simulink model "sampleModel196"  (Simulink 9.1)
settings: Solver=VariableStepAuto  StartTime=0.0  StopTime=10.0  RelTol=1e-3
undefined symbols (not defined in the file): DiscIntNeverNeededParam, Newton, Raphson
libraries: simulink x17
settings Model: Creator=DELL  LastModifiedBy=DELL
settings DataIOCC: SaveFormat=Dataset
settings OptimizationCC: LifeSpan=auto
settings DebuggingCC: UnderspecifiedInitializationDetection=Simplified  MergeDetectMultiDrivingBlocksExec=error  SFUnexpectedBacktrackingDiag=error  SFNoUnconditionalDefaultTransitionDiag=error  SFExecutionAtInitializationDiag=warning
settings HardwareCC: ProdBitPerPointer=64  ProdBitPerSizeT=64  ProdBitPerPtrDiffT=64  ProdLargestAtomicFloat=Float  ProdIntDivRoundTo=Zero  ProdEndianess=LittleEndian  ProdWordSize=64  ProdHWDeviceType=Intel->x86-64 (Windows64)
settings ModelReferenceCC: PropagateSignalLabelsOutOfModel=on
settings CodeAppCC: StateflowObjectComments=off
settings GRTTargetCC: TargetLangStandard=C99 (ISO)  CombineOutputUpdateFcns=on  GRTInterface=off
settings ConfigComp: CovMetricSettings=dwe  CovHtmlReporting=off  CovSaveCumulativeToWorkspaceVar=off  CovSaveSingleToWorkspaceVar=off  CovExternalEMLEnable=on

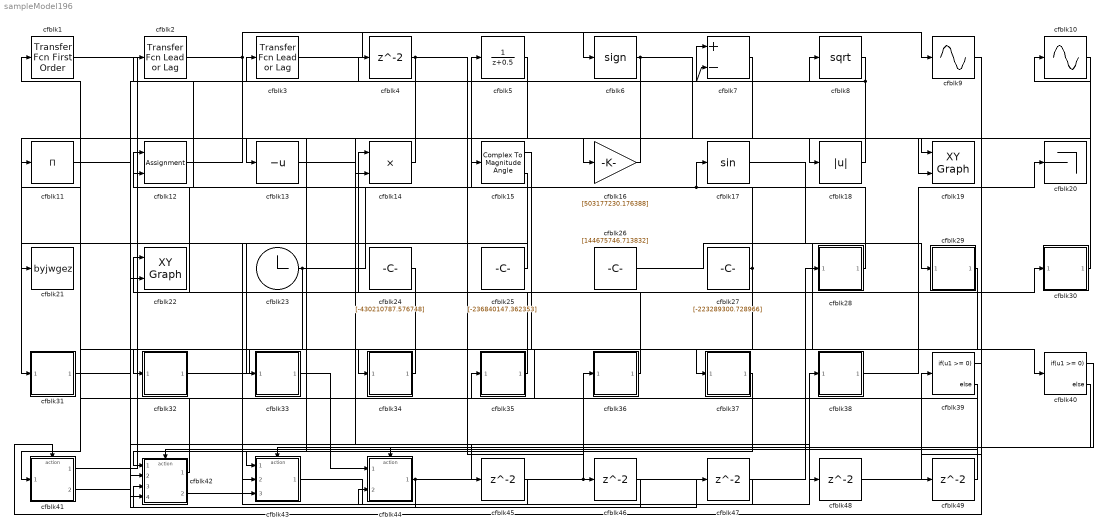
== system sampleModel196 ==
  cfblk1 : simulink/Discrete/Transfer Fcn First Order  PoleZ=0.95  ICPrevOutput=0.0  DoSatur=off
      settings: SourceProductName=Simulink
  cfblk10 : Sin  TimeSource=Use external signal  SampleTime=0
  cfblk11 : Product  Inputs=*
  cfblk12 : Assignment  DiagnosticForDimensions=Warning  IndexOptions=Index vector (dialog)  Indices=1  OutputSizes=1
  cfblk13 : UnaryMinus
  cfblk14 : Product  Inputs=**
  cfblk15 : ComplexToMagnitudeAngle
  cfblk16 : Gain  Gain=[503177230.176388]
  cfblk17 : Trigonometry
  cfblk18 : Abs
  cfblk19 : simulink/Sinks/XY Graph  xmin=-1  xmax=1  ymin=-1  ymax=1  st=-1
  cfblk2 : simulink/Discrete/Transfer Fcn Lead or Lag  PoleZ=0.95  ZeroZ=0.75  ICPrevOutput=0.0  ICPrevInput=0.0  DoSatur=off
      settings: SourceProductName=Simulink  SourceProductBaseCode=SL
  cfblk20 : Terminator
  cfblk21 : ToWorkspace  VariableName=byjwgez  SaveFormat=Timeseries  SampleTime=-1
  cfblk22 : simulink/Sinks/XY Graph  xmin=-1  xmax=1  ymin=-1  ymax=1  st=-1
  cfblk23 : Clock
  cfblk24 : Constant  Value=[-430210787.576748]  SampleTime=1
  cfblk25 : Constant  Value=[-236840147.362353]  SampleTime=1
  cfblk26 : Constant  Value=[144675746.713832]  SampleTime=1
  cfblk27 : Constant  Value=[-223289300.728966]  SampleTime=1
  cfblk28 : Subsystem
  cfblk29 : Subsystem
  cfblk3 : simulink/Discrete/Transfer Fcn Lead or Lag  PoleZ=0.95  ZeroZ=0.75  ICPrevOutput=0.0  ICPrevInput=0.0  DoSatur=off
      settings: SourceProductName=Simulink  SourceProductBaseCode=SL
  cfblk30 : Subsystem
  cfblk31 : Subsystem
  cfblk32 : Subsystem
  cfblk33 : Subsystem
  cfblk34 : Subsystem
  cfblk35 : Subsystem
  cfblk36 : Subsystem
  cfblk37 : Subsystem
  cfblk38 : Subsystem
  cfblk39 : If  IfExpression=u1 >= 0  SampleTime=1
  cfblk{4,45..49} (6 alike) : Delay  SampleTime=1
  cfblk40 : If  IfExpression=u1 >= 0  SampleTime=1
  cfblk41 : Subsystem  TreatAsAtomicUnit=on
  cfblk42 : Subsystem  TreatAsAtomicUnit=on
  cfblk43 : Subsystem  TreatAsAtomicUnit=on
  cfblk44 : Subsystem  TreatAsAtomicUnit=on
  cfblk5 : DiscreteTransferFcn  SampleTime=1
  cfblk6 : Signum
  cfblk7 : Sum  Inputs=+-
  cfblk8 : Sqrt  SaturateOnIntegerOverflow=on
  cfblk9 : Sin  TimeSource=Use external signal  SampleTime=0
  wires:
  cfblk33/1(cfblk2) -> cfblk44/1(cfblk1)
  cfblk15/1 -> cfblk34/1(cfblk1)
  cfblk43/1(cfblk2) -> cfblk38/1(cfblk1)
  cfblk27/1 -> cfblk35/1(cfblk1), cfblk12/2
  cfblk28/1(cfblk2) -> cfblk17/1, cfblk2/1
  cfblk26/1 -> cfblk40/1
  cfblk41/1(cfblk2) -> cfblk8/1
  cfblk23/1 -> cfblk5/1, cfblk42/4(cfblk13)
  cfblk8/1 -> cfblk18/1, cfblk7/2
  cfblk14/1 -> cfblk3/1
  cfblk6/1 -> cfblk13/1, cfblk19/2
  cfblk18/1 -> cfblk16/1
  cfblk17/1 -> cfblk29/1(cfblk1)
  cfblk4/1 -> cfblk31/1(cfblk1), cfblk46/1
  cfblk2/1 -> cfblk9/1, cfblk19/1
  cfblk3/1 -> cfblk6/1
  cfblk12/1 -> cfblk15/1
  cfblk16/1 -> cfblk4/1
  cfblk24/1 -> cfblk41/1(cfblk1)
  cfblk38/1(cfblk2) -> cfblk20/1
  cfblk5/1 -> cfblk43/1(cfblk1)
  cfblk30/1(cfblk2) -> cfblk10/1
  cfblk32/1(cfblk2) -> cfblk37/1(cfblk1)
  cfblk37/1(cfblk2) -> cfblk42/1(cfblk1)
  cfblk29/1(cfblk2) -> cfblk32/1(cfblk1)
  cfblk25/1 -> cfblk21/1
  cfblk34/1(cfblk2) -> cfblk22/1
  cfblk15/2 -> cfblk43/3(cfblk9)
  cfblk36/1(cfblk2) -> cfblk14/1
  cfblk7/1 -> cfblk22/2
  cfblk31/1(cfblk2) -> cfblk7/1
  cfblk44/1(cfblk2) -> cfblk28/1(cfblk1), cfblk36/1(cfblk1), cfblk42/3(cfblk12)
  cfblk10/1 -> cfblk14/2
  cfblk42/1(cfblk2) -> cfblk11/1
  cfblk42/2(cfblk14) -> cfblk30/1(cfblk1)
  cfblk1/1 -> cfblk33/1(cfblk1)
  cfblk35/1(cfblk2) -> cfblk12/1
  cfblk39/1 -> cfblk41/Action
  cfblk39/2 -> cfblk42/Action
  cfblk40/1 -> cfblk43/Action
  cfblk40/2 -> cfblk44/Action
  cfblk11/1 -> cfblk45/1
  cfblk45/1 -> cfblk43/2(cfblk8)
  cfblk46/1 -> cfblk42/2(cfblk11)
  cfblk41/2(cfblk13) -> cfblk47/1
  cfblk47/1 -> cfblk44/2(cfblk14)
  cfblk13/1 -> cfblk48/1
  cfblk48/1 -> cfblk39/1
  cfblk9/1 -> cfblk49/1
  cfblk49/1 -> cfblk1/1

== system sampleModel196/cfblk28 ==
  cfblk1 : Inport
  cfblk2 : Outport
  wires:
  cfblk1/1 -> cfblk2/1

== system sampleModel196/cfblk29 ==
  cfblk1 : Inport
  cfblk2 : Outport
  wires:
  cfblk1/1 -> cfblk2/1

== system sampleModel196/cfblk30 ==
  cfblk1 : Inport
  cfblk2 : Outport
  wires:
  cfblk1/1 -> cfblk2/1

== system sampleModel196/cfblk31 ==
  cfblk1 : Inport
  cfblk2 : Outport
  wires:
  cfblk1/1 -> cfblk2/1

== system sampleModel196/cfblk32 ==
  cfblk1 : Inport
  cfblk2 : Outport
  wires:
  cfblk1/1 -> cfblk2/1

== system sampleModel196/cfblk33 ==
  cfblk1 : Inport
  cfblk2 : Outport
  wires:
  cfblk1/1 -> cfblk2/1

== system sampleModel196/cfblk34 ==
  cfblk1 : Inport
  cfblk2 : Outport
  wires:
  cfblk1/1 -> cfblk2/1

== system sampleModel196/cfblk35 ==
  cfblk1 : Inport
  cfblk2 : Outport
  wires:
  cfblk1/1 -> cfblk2/1

== system sampleModel196/cfblk36 ==
  cfblk1 : Inport
  cfblk2 : Outport
  wires:
  cfblk1/1 -> cfblk2/1

== system sampleModel196/cfblk37 ==
  cfblk1 : Inport
  cfblk2 : Outport
  wires:
  cfblk1/1 -> cfblk2/1

== system sampleModel196/cfblk38 ==
  cfblk1 : Inport
  cfblk2 : Outport
  wires:
  cfblk1/1 -> cfblk2/1

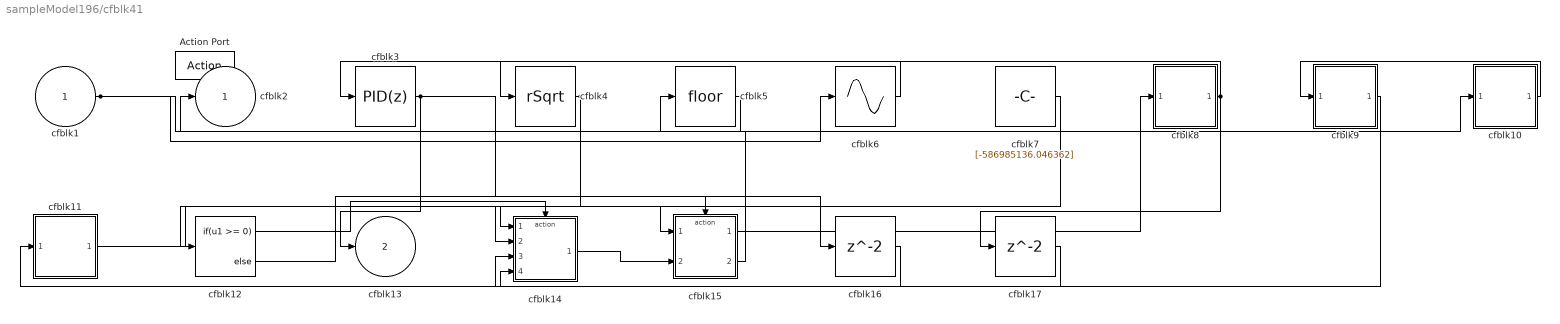
== system sampleModel196/cfblk41 ==
  cfblk1 : Inport
  Action Port : ActionPort  ActionType=then
  cfblk10 : Subsystem
  cfblk11 : Subsystem
  cfblk12 : If  IfExpression=u1 >= 0  SampleTime=1
  cfblk14 : Subsystem  TreatAsAtomicUnit=on
  cfblk15 : Subsystem  TreatAsAtomicUnit=on
  cfblk16 : Delay
  cfblk17 : Delay
  cfblk3 : simulink/Continuous/PID Controller  Controller=PID  TimeDomain=Discrete-time  SampleTime=-1  IntegratorMethod=Forward Euler  FilterMethod=Forward Euler  Form=Parallel  UseFilter=on  ControllerParametersSource=internal  P=1  I=1  D=0  N=100  InitialConditionSource=internal  InitialConditionForIntegrator=0  InitialConditionForFilter=0  ExternalReset=none  LimitOutput=off  UpperSaturationLimit=inf  LowerSaturationLimit=-inf  LinearizeAsGain=off  AntiWindupMode=none  Kb=1  TrackingMode=off  Kt=1  PParamMin=[]  PParamMax=[]  IParamMin=[]  IParamMax=[]  DParamMin=[]  DParamMax=[]  NParamMin=[]  NParamMax=[]  KbParamMin=[]  KbParamMax=[]  KtParamMin=[]  KtParamMax=[]  POutMin=[]  POutMax=[]  IOutMin=[]  IOutMax=[]  DOutMin=[]  DOutMax=[]  NOutMin=[]  NOutMax=[]  KbOutMin=[]  KbOutMax=[]  KtOutMin=[]  KtOutMax=[]  IntegratorOutMin=[]  IntegratorOutMax=[]  FilterOutMin=[]  FilterOutMax=[]  SumOutMin=[]  SumOutMax=[]  SumI1OutMin=[]  SumI1OutMax=[]  SumI2OutMin=[]  SumI2OutMax=[]  SumI3OutMin=[]  SumI3OutMax=[]  SumDOutMin=[]  SumDOutMax=[]  SaturationOutMin=[]  SaturationOutMax=[]  IntegratorContinuousStateAttributes=''  IntegratorStateMustResolveToSignalObject=off  IntegratorRTWStateStorageClass=Auto  FilterContinuousStateAttributes=''  FilterStateMustResolveToSignalObject=off  FilterRTWStateStorageClass=Auto  DifferentiatorICPrevScaledInput=0  DifferentiatorOutMin=[]  DifferentiatorOutMax=[]  FilterDiffOutCoefMin=[]  FilterDiffOutCoefMax=[]  SumDenOutMin=[]  SumDenOutMax=[]  SumNumOutMin=[]  SumNumOutMax=[]  ReciprocalOutMin=[]  ReciprocalOutMax=[]  DivideOutMin=[]  DivideOutMax=[]  TunerSelectOption=Transfer Function Based (PID Tuner App)
  cfblk4 : Sqrt  Operator=rSqrt  AlgorithmType=Newton-Raphson  SaturateOnIntegerOverflow=on
  cfblk5 : Rounding
  cfblk6 : Sin  TimeSource=Use external signal  SampleTime=0
  cfblk7 : Constant  Value=[-586985136.046362]  SampleTime=1
  cfblk8 : Subsystem
  cfblk9 : Subsystem
  cfblk2 : Outport
  cfblk13 : Outport  Port=2
  wires:
  cfblk15/1(cfblk2) -> cfblk8/1(cfblk1)
  cfblk8/1(cfblk2) -> cfblk3/1, cfblk17/1
  cfblk5/1 -> cfblk2/1
  cfblk9/1(cfblk2) -> cfblk11/1(cfblk1)
  cfblk11/1(cfblk2) -> cfblk15/1(cfblk1)
  cfblk7/1 -> cfblk14/1(cfblk1)
  cfblk1/1 -> cfblk6/1, cfblk10/1(cfblk1)
  cfblk3/1 -> cfblk13/1, cfblk16/1
  cfblk4/1 -> cfblk12/1, cfblk14/2(cfblk11)
  cfblk6/1 -> cfblk4/1
  cfblk10/1(cfblk2) -> cfblk9/1(cfblk1)
  cfblk15/2(cfblk9) -> cfblk5/1
  cfblk14/1(cfblk2) -> cfblk15/2(cfblk8)
  cfblk12/1 -> cfblk14/Action
  cfblk12/2 -> cfblk15/Action
  cfblk16/1 -> cfblk14/4(cfblk13)
  cfblk17/1 -> cfblk14/3(cfblk12)

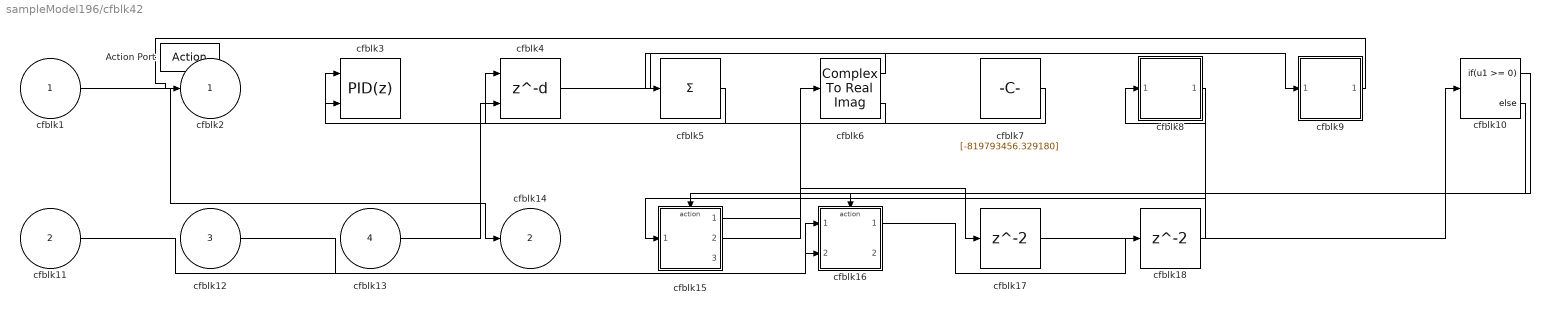
== system sampleModel196/cfblk42 ==
  cfblk1 : Inport
  cfblk11 : Inport  Port=2
  cfblk12 : Inport  Port=3
  cfblk13 : Inport  Port=4
  Action Port : ActionPort  ActionType=else
  cfblk10 : If  IfExpression=u1 >= 0  SampleTime=1
  cfblk15 : Subsystem  TreatAsAtomicUnit=on
  cfblk16 : Subsystem  TreatAsAtomicUnit=on
  cfblk17 : Delay
  cfblk18 : Delay
  cfblk3 : simulink/Continuous/PID Controller (2DOF)  Controller=PID  TimeDomain=Discrete-time  SampleTime=-1  IntegratorMethod=Forward Euler  FilterMethod=Forward Euler  Form=Parallel  UseFilter=on  ControllerParametersSource=internal  P=1  I=1  D=0  N=100  b=1  c=1  InitialConditionSource=internal  InitialConditionForIntegrator=0  InitialConditionForFilter=0  ExternalReset=none  LimitOutput=off  UpperSaturationLimit=inf  LowerSaturationLimit=-inf  LinearizeAsGain=off  AntiWindupMode=none  Kb=1  TrackingMode=off  Kt=1  PParamMin=[]  PParamMax=[]  IParamMin=[]  IParamMax=[]  DParamMin=[]  DParamMax=[]  NParamMin=[]  NParamMax=[]  bParamMin=[]  bParamMax=[]  cParamMin=[]  cParamMax=[]  KbParamMin=[]  KbParamMax=[]  KtParamMin=[]  KtParamMax=[]  POutMin=[]  POutMax=[]  IOutMin=[]  IOutMax=[]  DOutMin=[]  DOutMax=[]  NOutMin=[]  NOutMax=[]  bOutMin=[]  bOutMax=[]  cOutMin=[]  cOutMax=[]  KbOutMin=[]  KbOutMax=[]  KtOutMin=[]  KtOutMax=[]  IntegratorOutMin=[]  IntegratorOutMax=[]  FilterOutMin=[]  FilterOutMax=[]  SumOutMin=[]  SumOutMax=[]  Sum1OutMin=[]  Sum1OutMax=[]  Sum2OutMin=[]  Sum2OutMax=[]  Sum3OutMin=[]  Sum3OutMax=[]  SumI1OutMin=[]  SumI1OutMax=[]  SumI2OutMin=[]  SumI2OutMax=[]  SumI3OutMin=[]  SumI3OutMax=[]  SumDOutMin=[]  SumDOutMax=[]  SaturationOutMin=[]  SaturationOutMax=[]  IntegratorContinuousStateAttributes=''  IntegratorStateMustResolveToSignalObject=off  IntegratorRTWStateStorageClass=Auto  FilterContinuousStateAttributes=''  FilterStateMustResolveToSignalObject=off  FilterRTWStateStorageClass=Auto  DifferentiatorICPrevScaledInput=0  DifferentiatorOutMin=[]  DifferentiatorOutMax=[]  FilterDiffOutCoefMin=[]  FilterDiffOutCoefMax=[]  SumDenOutMin=[]  SumDenOutMax=[]  SumNumOutMin=[]  SumNumOutMax=[]  ReciprocalOutMin=[]  ReciprocalOutMax=[]  DivideOutMin=[]  DivideOutMax=[]  TunerSelectOption=Transfer Function Based (PID Tuner App)
  cfblk4 : Delay  DelayLengthSource=Input port
      settings: InputPortMap=u0,p1
  cfblk5 : Sum  Inputs=+
  cfblk6 : ComplexToRealImag
  cfblk7 : Constant  Value=[-819793456.329180]  SampleTime=1
  cfblk8 : Subsystem
  cfblk9 : Subsystem
  cfblk2 : Outport
  cfblk14 : Outport  Port=2
  wires:
  cfblk4/1 -> cfblk9/1(cfblk1)
  cfblk1/1 -> cfblk14/1
  cfblk11/1 -> cfblk16/1(cfblk1)
  cfblk7/1 -> cfblk4/1
  cfblk9/1(cfblk2) -> cfblk2/1
  cfblk12/1 -> cfblk16/2(cfblk11)
  cfblk6/1 -> cfblk5/1
  cfblk13/1 -> cfblk4/2
  cfblk8/1(cfblk2) -> cfblk15/1(cfblk1)
  cfblk6/2 -> cfblk3/1
  cfblk15/2(cfblk16) -> cfblk6/1
  cfblk5/1 -> cfblk3/2
  cfblk10/1 -> cfblk15/Action
  cfblk10/2 -> cfblk16/Action
  cfblk15/1(cfblk2) -> cfblk17/1
  cfblk17/1 -> cfblk10/1
  cfblk16/1(cfblk2) -> cfblk18/1
  cfblk18/1 -> cfblk8/1(cfblk1)

== system sampleModel196/cfblk43 ==
  cfblk1 : Inport
  cfblk8 : Inport  Port=2
  cfblk9 : Inport  Port=3
  Action Port : ActionPort  ActionType=then
  cfblk3 : DiscreteStateSpace  SampleTime=-1
  cfblk4 : DiscreteFilter
  cfblk5 : DiscreteZeroPole  Poles=[0 0.5]  Gain=1  SampleTime=-1
  cfblk6 : Constant  Value=[-475565543.118266]  SampleTime=1
  cfblk7 : Subsystem
  cfblk2 : Outport
  wires:
  cfblk4/1 -> cfblk2/1
  cfblk6/1 -> cfblk4/1
  cfblk8/1 -> cfblk5/1
  cfblk5/1 -> cfblk7/1(cfblk1)
  cfblk7/1(cfblk2) -> cfblk3/1

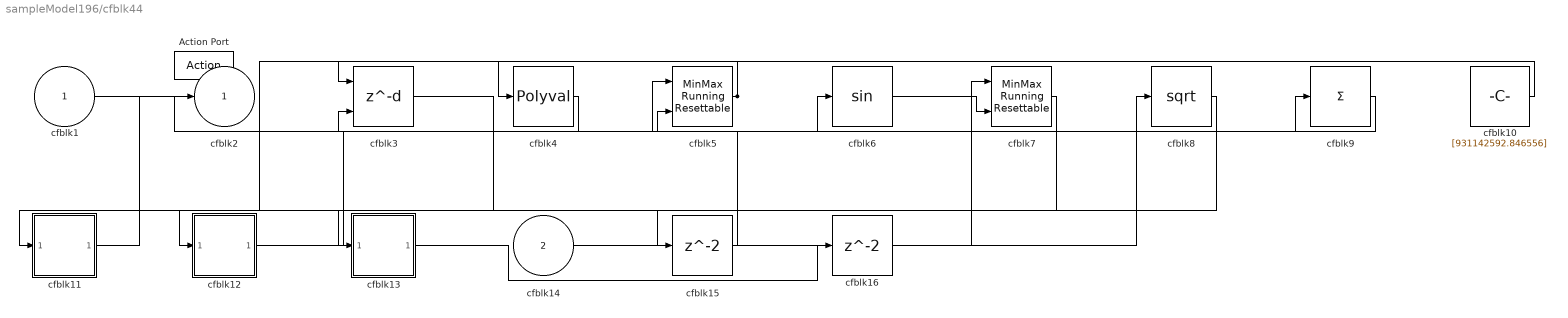
== system sampleModel196/cfblk44 ==
  cfblk1 : Inport
  cfblk14 : Inport  Port=2
  Action Port : ActionPort  ActionType=else
  cfblk10 : Constant  Value=[931142592.846556]  SampleTime=1
  cfblk11 : Subsystem
  cfblk12 : Subsystem
  cfblk13 : Subsystem
  cfblk15 : Delay
  cfblk16 : Delay
  cfblk3 : Delay  DelayLengthSource=Input port
      settings: InputPortMap=u0,p1
  cfblk4 : Polyval  Coefs=[ +2.081618890e-019, -1.441693666e-014, +4.719686976e-010, -8.536869453e-006, +1.621573104e-001, -8.087801117e+001 ]
  cfblk5 : simulink/Math Operations/MinMax Running Resettable  Function=min  vinit=0.0
  cfblk6 : Trigonometry
  cfblk7 : simulink/Math Operations/MinMax Running Resettable  Function=min  vinit=0.0
  cfblk8 : Sqrt  SaturateOnIntegerOverflow=on
  cfblk9 : Sum  Inputs=+
  cfblk2 : Outport
  wires:
  cfblk12/1(cfblk2) -> cfblk6/1
  cfblk10/1 -> cfblk12/1(cfblk1)
  cfblk11/1(cfblk2) -> cfblk2/1
  cfblk1/1 -> cfblk9/1
  cfblk14/1 -> cfblk8/1
  cfblk5/1 -> cfblk3/1, cfblk4/1
  cfblk9/1 -> cfblk5/2
  cfblk4/1 -> cfblk3/2
  cfblk7/1 -> cfblk13/1(cfblk1)
  cfblk6/1 -> cfblk7/2
  cfblk8/1 -> cfblk11/1(cfblk1)
  cfblk3/1 -> cfblk15/1
  cfblk15/1 -> cfblk5/1
  cfblk13/1(cfblk2) -> cfblk16/1
  cfblk16/1 -> cfblk7/1

== system sampleModel196/cfblk41/cfblk10 ==
  cfblk1 : Inport
  cfblk2 : Outport
  wires:
  cfblk1/1 -> cfblk2/1

== system sampleModel196/cfblk41/cfblk11 ==
  cfblk1 : Inport
  cfblk2 : Outport
  wires:
  cfblk1/1 -> cfblk2/1

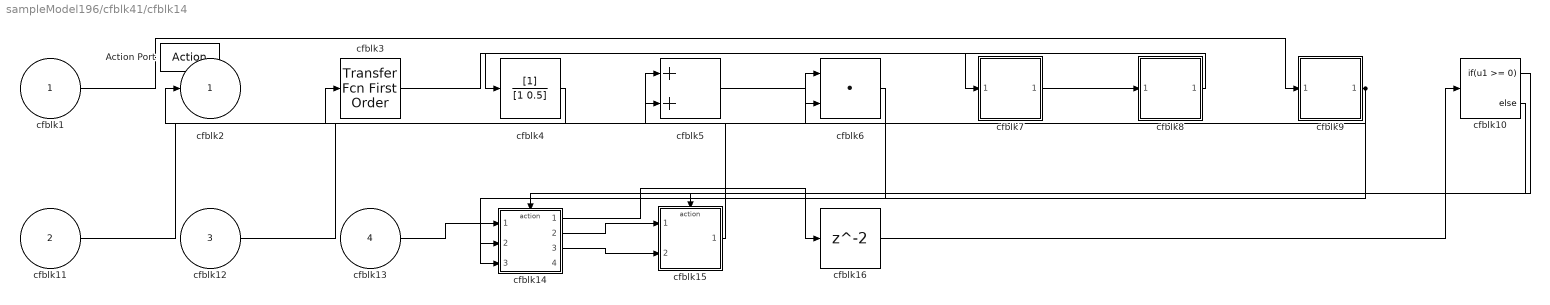
== system sampleModel196/cfblk41/cfblk14 ==
  cfblk1 : Inport
  cfblk11 : Inport  Port=2
  cfblk12 : Inport  Port=3
  cfblk13 : Inport  Port=4
  Action Port : ActionPort  ActionType=then
  cfblk10 : If  IfExpression=u1 >= 0  SampleTime=1
  cfblk14 : Subsystem  TreatAsAtomicUnit=on
  cfblk15 : Subsystem  TreatAsAtomicUnit=on
  cfblk16 : Delay
  cfblk3 : simulink/Discrete/Transfer Fcn First Order  PoleZ=0.95  ICPrevOutput=0.0  DoSatur=off
      settings: SourceProductName=Simulink
  cfblk4 : DiscreteFilter
  cfblk5 : Sum
  cfblk6 : DotProduct  InputSameDT=on  OutDataTypeStr=Inherit: Inherit via internal rule
  cfblk7 : Subsystem
  cfblk8 : Subsystem
  cfblk9 : Subsystem
  cfblk2 : Outport
  wires:
  cfblk8/1(cfblk2) -> cfblk4/1
  cfblk11/1 -> cfblk6/1
  cfblk1/1 -> cfblk9/1(cfblk1)
  cfblk12/1 -> cfblk5/1
  cfblk15/1(cfblk2) -> cfblk3/1
  cfblk3/1 -> cfblk7/1(cfblk1)
  cfblk9/1(cfblk2) -> cfblk5/2, cfblk14/3(cfblk13)
  cfblk5/1 -> cfblk6/2
  cfblk7/1(cfblk2) -> cfblk8/1(cfblk1)
  cfblk13/1 -> cfblk14/1(cfblk1)
  cfblk4/1 -> cfblk2/1
  cfblk6/1 -> cfblk14/2(cfblk12)
  cfblk14/2(cfblk14) -> cfblk15/1(cfblk1)
  cfblk14/3(cfblk15) -> cfblk15/2(cfblk16)
  cfblk10/1 -> cfblk14/Action
  cfblk10/2 -> cfblk15/Action
  cfblk14/1(cfblk2) -> cfblk16/1
  cfblk16/1 -> cfblk10/1

== system sampleModel196/cfblk41/cfblk15 ==
  cfblk1 : Inport
  cfblk8 : Inport  Port=2
  Action Port : ActionPort  ActionType=else
  cfblk3 : DiscreteFir
  cfblk4 : simulink/Discrete/Difference  ICPrevInput=0.0  OutMin=[]  OutMax=[]  OutDataTypeStr=Inherit: Inherit via back propagation  OutDataType=fixdt(1, 16)  OutScaling=2^-10  DoSatur=off
  cfblk5 : Constant  Value=[-973339246.254504]  SampleTime=1
  cfblk6 : Constant  Value=[-836028439.478681]  SampleTime=1
  cfblk7 : Constant  Value=[-477392529.505172]  SampleTime=1
  cfblk2 : Outport
  cfblk9 : Outport  Port=2
  wires:
  cfblk7/1 -> cfblk3/1
  cfblk8/1 -> cfblk4/1
  cfblk1/1 -> cfblk2/1
  cfblk3/1 -> cfblk9/1

== system sampleModel196/cfblk41/cfblk8 ==
  cfblk1 : Inport
  cfblk2 : Outport
  wires:
  cfblk1/1 -> cfblk2/1

== system sampleModel196/cfblk41/cfblk9 ==
  cfblk1 : Inport
  cfblk2 : Outport
  wires:
  cfblk1/1 -> cfblk2/1

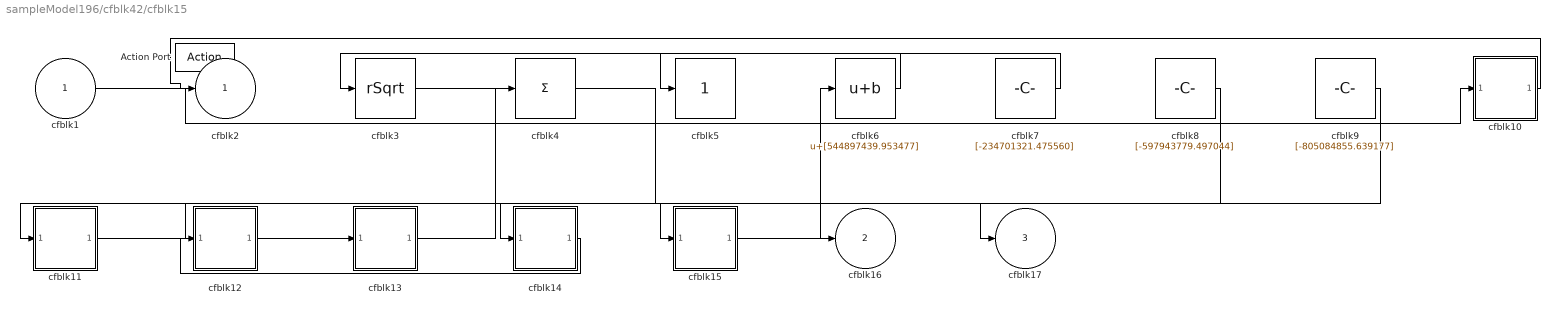
== system sampleModel196/cfblk42/cfblk15 ==
  cfblk1 : Inport
  Action Port : ActionPort  ActionType=then
  cfblk10 : Subsystem
  cfblk11 : Subsystem
  cfblk12 : Subsystem
  cfblk13 : Subsystem
  cfblk14 : Subsystem
  cfblk15 : Subsystem
  cfblk3 : Sqrt  Operator=rSqrt  AlgorithmType=Newton-Raphson  SaturateOnIntegerOverflow=on
  cfblk4 : Sum  Inputs=+
  cfblk5 : simulink/Math Operations/Slider Gain  gain=1  low=0  high=2
  cfblk6 : Bias  Bias=[544897439.953477]
  cfblk7 : Constant  Value=[-234701321.475560]  SampleTime=1
  cfblk8 : Constant  Value=[-597943779.497044]  SampleTime=1
  cfblk9 : Constant  Value=[-805084855.639177]  SampleTime=1
  cfblk2 : Outport
  cfblk16 : Outport  Port=2
  cfblk17 : Outport  Port=3
  wires:
  cfblk1/1 -> cfblk10/1(cfblk1)
  cfblk8/1 -> cfblk14/1(cfblk1)
  cfblk15/1(cfblk2) -> cfblk6/1
  cfblk7/1 -> cfblk3/1
  cfblk13/1(cfblk2) -> cfblk4/1
  cfblk11/1(cfblk2) -> cfblk16/1
  cfblk14/1(cfblk2) -> cfblk12/1(cfblk1)
  cfblk10/1(cfblk2) -> cfblk2/1
  cfblk12/1(cfblk2) -> cfblk13/1(cfblk1)
  cfblk6/1 -> cfblk5/1
  cfblk4/1 -> cfblk17/1
  cfblk9/1 -> cfblk11/1(cfblk1)
  cfblk3/1 -> cfblk15/1(cfblk1)

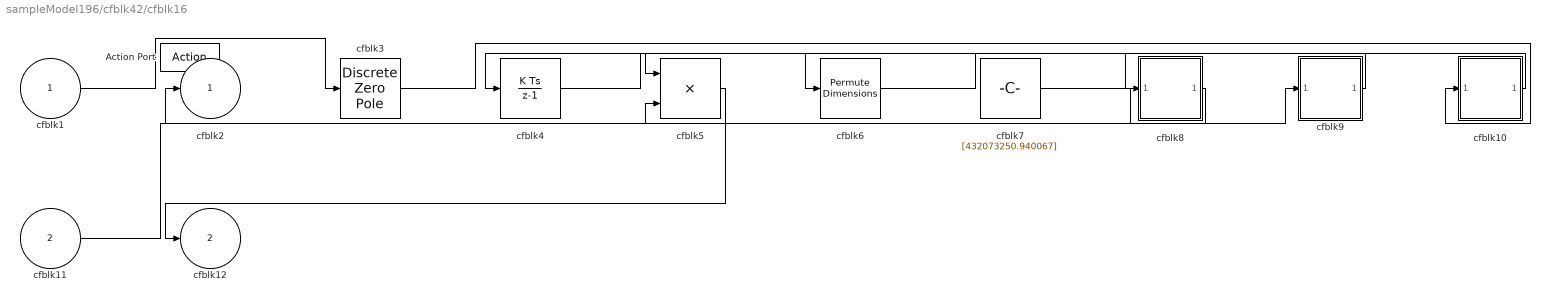
== system sampleModel196/cfblk42/cfblk16 ==
  cfblk1 : Inport
  cfblk11 : Inport  Port=2
  Action Port : ActionPort  ActionType=else
  cfblk10 : Subsystem
  cfblk3 : DiscreteZeroPole  Poles=[0 0.5]  Gain=1  SampleTime=-1
  cfblk4 : DiscreteIntegrator  SampleTime=-1  ICPrevOutput=DiscIntNeverNeededParam  ICPrevScaledInput=DiscIntNeverNeededParam
  cfblk5 : Product
  cfblk6 : PermuteDimensions
  cfblk7 : Constant  Value=[432073250.940067]  SampleTime=1
  cfblk8 : Subsystem
  cfblk9 : Subsystem
  cfblk2 : Outport
  cfblk12 : Outport  Port=2
  wires:
  cfblk5/1 -> cfblk12/1
  cfblk10/1(cfblk2) -> cfblk4/1
  cfblk7/1 -> cfblk9/1(cfblk1)
  cfblk9/1(cfblk2) -> cfblk5/1
  cfblk8/1(cfblk2) -> cfblk2/1
  cfblk1/1 -> cfblk3/1
  cfblk11/1 -> cfblk5/2
  cfblk3/1 -> cfblk10/1(cfblk1)
  cfblk6/1 -> cfblk8/1(cfblk1)
  cfblk4/1 -> cfblk6/1

== system sampleModel196/cfblk42/cfblk8 ==
  cfblk1 : Inport
  cfblk2 : Outport
  wires:
  cfblk1/1 -> cfblk2/1

== system sampleModel196/cfblk42/cfblk9 ==
  cfblk1 : Inport
  cfblk2 : Outport
  wires:
  cfblk1/1 -> cfblk2/1

== system sampleModel196/cfblk43/cfblk7 ==
  cfblk1 : Inport
  cfblk2 : Outport
  wires:
  cfblk1/1 -> cfblk2/1

== system sampleModel196/cfblk44/cfblk11 ==
  cfblk1 : Inport
  cfblk2 : Outport
  wires:
  cfblk1/1 -> cfblk2/1

== system sampleModel196/cfblk44/cfblk12 ==
  cfblk1 : Inport
  cfblk2 : Outport
  wires:
  cfblk1/1 -> cfblk2/1

== system sampleModel196/cfblk44/cfblk13 ==
  cfblk1 : Inport
  cfblk2 : Outport
  wires:
  cfblk1/1 -> cfblk2/1

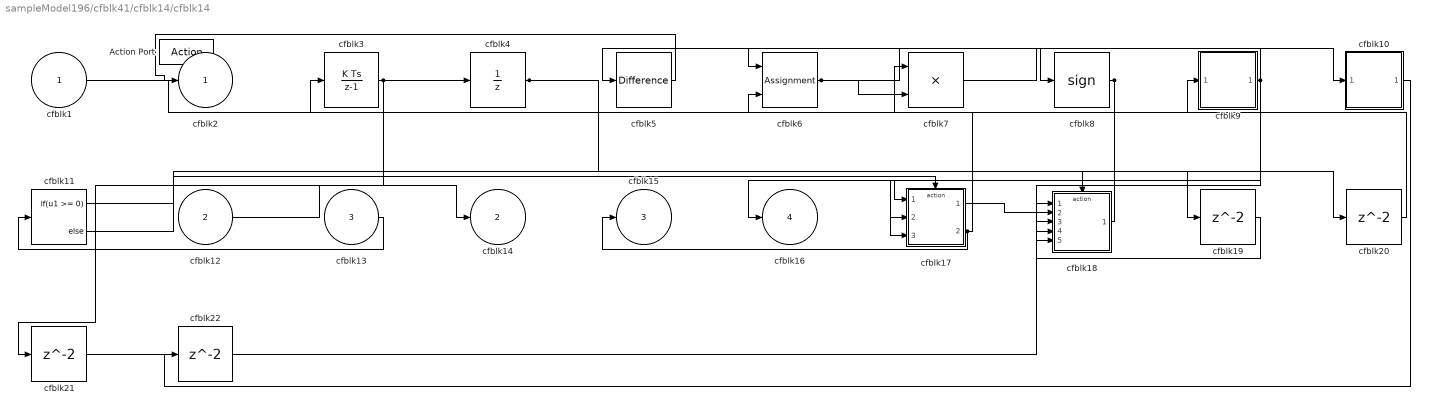
== system sampleModel196/cfblk41/cfblk14/cfblk14 ==
  cfblk1 : Inport
  cfblk12 : Inport  Port=2
  cfblk13 : Inport  Port=3
  Action Port : ActionPort  ActionType=then
  cfblk10 : Subsystem
  cfblk11 : If  IfExpression=u1 >= 0  SampleTime=1
  cfblk17 : Subsystem  TreatAsAtomicUnit=on
  cfblk18 : Subsystem  TreatAsAtomicUnit=on
  cfblk{19..22} (4 alike) : Delay
  cfblk3 : DiscreteIntegrator  SampleTime=-1  ICPrevOutput=DiscIntNeverNeededParam  ICPrevScaledInput=DiscIntNeverNeededParam
  cfblk4 : UnitDelay  SampleTime=-1
  cfblk5 : simulink/Discrete/Difference  ICPrevInput=0.0  OutMin=[]  OutMax=[]  OutDataTypeStr=Inherit: Inherit via back propagation  OutDataType=fixdt(1, 16)  OutScaling=2^-10  DoSatur=off
  cfblk6 : Assignment  DiagnosticForDimensions=Warning  IndexOptions=Index vector (dialog)  Indices=1  OutputSizes=1
  cfblk7 : Product  Inputs=**
  cfblk8 : Signum
  cfblk9 : Subsystem
  cfblk2 : Outport
  cfblk14 : Outport  Port=2
  cfblk15 : Outport  Port=3
  cfblk16 : Outport  Port=4
  wires:
  cfblk1/1 -> cfblk9/1(cfblk1)
  cfblk5/1 -> cfblk2/1
  cfblk9/1(cfblk2) -> cfblk6/1, cfblk5/1, cfblk17/2(cfblk7), cfblk18/5(cfblk10)
  cfblk3/1 -> cfblk4/1, cfblk21/1
  cfblk17/1(cfblk2) -> cfblk18/2(cfblk7)
  cfblk12/1 -> cfblk14/1
  cfblk4/1 -> cfblk19/1, cfblk20/1
  cfblk8/1 -> cfblk17/1(cfblk1), cfblk17/3(cfblk8), cfblk16/1
  cfblk6/1 -> cfblk8/1, cfblk7/2
  cfblk18/1(cfblk2) -> cfblk3/1
  cfblk13/1 -> cfblk11/1
  cfblk17/2(cfblk9) -> cfblk7/1, cfblk15/1
  cfblk7/1 -> cfblk10/1(cfblk1)
  cfblk11/1 -> cfblk17/Action
  cfblk11/2 -> cfblk18/Action
  cfblk19/1 -> cfblk18/3(cfblk8)
  cfblk20/1 -> cfblk6/2
  cfblk21/1 -> cfblk18/4(cfblk9)
  cfblk10/1(cfblk2) -> cfblk22/1
  cfblk22/1 -> cfblk18/1(cfblk1)

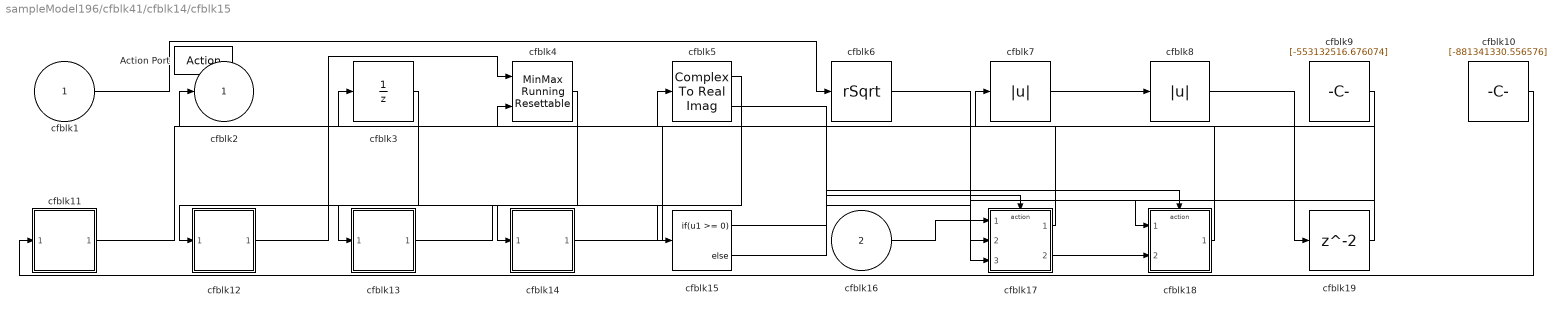
== system sampleModel196/cfblk41/cfblk14/cfblk15 ==
  cfblk1 : Inport
  cfblk16 : Inport  Port=2
  Action Port : ActionPort  ActionType=else
  cfblk10 : Constant  Value=[-881341330.556576]  SampleTime=1
  cfblk11 : Subsystem
  cfblk12 : Subsystem
  cfblk13 : Subsystem
  cfblk14 : Subsystem
  cfblk15 : If  IfExpression=u1 >= 0  SampleTime=1
  cfblk17 : Subsystem  TreatAsAtomicUnit=on
  cfblk18 : Subsystem  TreatAsAtomicUnit=on
  cfblk19 : Delay
  cfblk3 : UnitDelay  SampleTime=-1
  cfblk4 : simulink/Math Operations/MinMax Running Resettable  Function=min  vinit=0.0
  cfblk5 : ComplexToRealImag
  cfblk6 : Sqrt  Operator=rSqrt  AlgorithmType=Newton-Raphson  SaturateOnIntegerOverflow=on
  cfblk7 : Abs
  cfblk8 : Abs
  cfblk9 : Constant  Value=[-553132516.676074]  SampleTime=1
  cfblk2 : Outport
  wires:
  cfblk17/1(cfblk2) -> cfblk3/1
  cfblk4/1 -> cfblk14/1(cfblk1)
  cfblk14/1(cfblk2) -> cfblk7/1
  cfblk12/1(cfblk2) -> cfblk4/1
  cfblk6/1 -> cfblk18/1(cfblk1)
  cfblk3/1 -> cfblk12/1(cfblk1)
  cfblk7/1 -> cfblk8/1
  cfblk16/1 -> cfblk17/1(cfblk1)
  cfblk1/1 -> cfblk6/1
  cfblk17/2(cfblk17) -> cfblk18/2(cfblk7)
  cfblk10/1 -> cfblk11/1(cfblk1)
  cfblk13/1(cfblk2) -> cfblk15/1
  cfblk18/1(cfblk2) -> cfblk2/1
  cfblk5/1 -> cfblk13/1(cfblk1)
  cfblk5/2 -> cfblk17/2(cfblk15)
  cfblk11/1(cfblk2) -> cfblk5/1
  cfblk9/1 -> cfblk17/3(cfblk16)
  cfblk15/1 -> cfblk17/Action
  cfblk15/2 -> cfblk18/Action
  cfblk8/1 -> cfblk19/1
  cfblk19/1 -> cfblk4/2

== system sampleModel196/cfblk41/cfblk14/cfblk7 ==
  cfblk1 : Inport
  cfblk2 : Outport
  wires:
  cfblk1/1 -> cfblk2/1

== system sampleModel196/cfblk41/cfblk14/cfblk8 ==
  cfblk1 : Inport
  cfblk2 : Outport
  wires:
  cfblk1/1 -> cfblk2/1

== system sampleModel196/cfblk41/cfblk14/cfblk9 ==
  cfblk1 : Inport
  cfblk2 : Outport
  wires:
  cfblk1/1 -> cfblk2/1

== system sampleModel196/cfblk42/cfblk15/cfblk10 ==
  cfblk1 : Inport
  cfblk2 : Outport
  wires:
  cfblk1/1 -> cfblk2/1

== system sampleModel196/cfblk42/cfblk15/cfblk11 ==
  cfblk1 : Inport
  cfblk2 : Outport
  wires:
  cfblk1/1 -> cfblk2/1

== system sampleModel196/cfblk42/cfblk15/cfblk12 ==
  cfblk1 : Inport
  cfblk2 : Outport
  wires:
  cfblk1/1 -> cfblk2/1

== system sampleModel196/cfblk42/cfblk15/cfblk13 ==
  cfblk1 : Inport
  cfblk2 : Outport
  wires:
  cfblk1/1 -> cfblk2/1

== system sampleModel196/cfblk42/cfblk15/cfblk14 ==
  cfblk1 : Inport
  cfblk2 : Outport
  wires:
  cfblk1/1 -> cfblk2/1

== system sampleModel196/cfblk42/cfblk15/cfblk15 ==
  cfblk1 : Inport
  cfblk2 : Outport
  wires:
  cfblk1/1 -> cfblk2/1

== system sampleModel196/cfblk42/cfblk16/cfblk10 ==
  cfblk1 : Inport
  cfblk2 : Outport
  wires:
  cfblk1/1 -> cfblk2/1

== system sampleModel196/cfblk42/cfblk16/cfblk8 ==
  cfblk1 : Inport
  cfblk2 : Outport
  wires:
  cfblk1/1 -> cfblk2/1

== system sampleModel196/cfblk42/cfblk16/cfblk9 ==
  cfblk1 : Inport
  cfblk2 : Outport
  wires:
  cfblk1/1 -> cfblk2/1

== system sampleModel196/cfblk41/cfblk14/cfblk14/cfblk10 ==
  cfblk1 : Inport
  cfblk2 : Outport
  wires:
  cfblk1/1 -> cfblk2/1

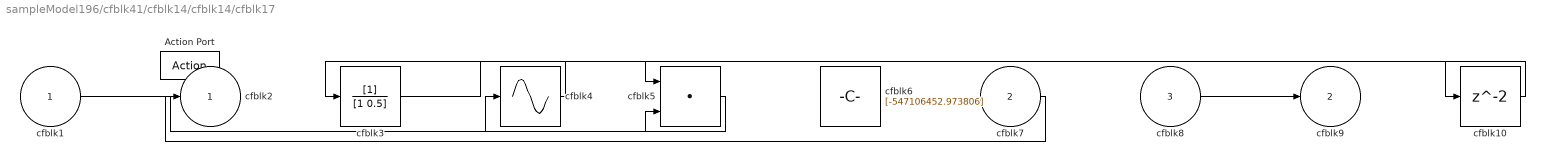
== system sampleModel196/cfblk41/cfblk14/cfblk14/cfblk17 ==
  cfblk1 : Inport
  cfblk7 : Inport  Port=2
  cfblk8 : Inport  Port=3
  Action Port : ActionPort  ActionType=then
  cfblk10 : Delay
  cfblk3 : DiscreteFilter
  cfblk4 : Sin  TimeSource=Use external signal  SampleTime=0
  cfblk5 : DotProduct  InputSameDT=on  OutDataTypeStr=Inherit: Inherit via internal rule
  cfblk6 : Constant  Value=[-547106452.973806]  SampleTime=1
  cfblk2 : Outport
  cfblk9 : Outport  Port=2
  wires:
  cfblk8/1 -> cfblk9/1
  cfblk5/1 -> cfblk4/1
  cfblk1/1 -> cfblk5/2
  cfblk7/1 -> cfblk2/1
  cfblk4/1 -> cfblk3/1
  cfblk3/1 -> cfblk10/1
  cfblk10/1 -> cfblk5/1

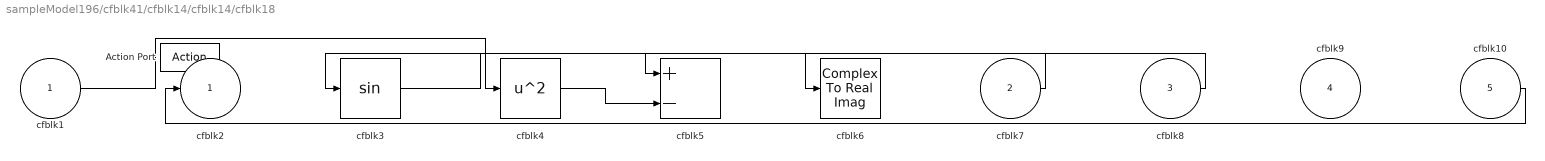
== system sampleModel196/cfblk41/cfblk14/cfblk14/cfblk18 ==
  cfblk1 : Inport
  cfblk7 : Inport  Port=2
  cfblk8 : Inport  Port=3
  cfblk9 : Inport  Port=4
  cfblk10 : Inport  Port=5
  Action Port : ActionPort  ActionType=else
  cfblk3 : Trigonometry
  cfblk4 : Math  Operator=square  SaturateOnIntegerOverflow=on
  cfblk5 : Sum  Inputs=+-
  cfblk6 : ComplexToRealImag
  cfblk2 : Outport
  wires:
  cfblk10/1 -> cfblk2/1
  cfblk1/1 -> cfblk4/1
  cfblk3/1 -> cfblk6/1
  cfblk7/1 -> cfblk3/1
  cfblk8/1 -> cfblk5/1
  cfblk4/1 -> cfblk5/2

== system sampleModel196/cfblk41/cfblk14/cfblk14/cfblk9 ==
  cfblk1 : Inport
  cfblk2 : Outport
  wires:
  cfblk1/1 -> cfblk2/1

== system sampleModel196/cfblk41/cfblk14/cfblk15/cfblk11 ==
  cfblk1 : Inport
  cfblk2 : Outport
  wires:
  cfblk1/1 -> cfblk2/1

== system sampleModel196/cfblk41/cfblk14/cfblk15/cfblk12 ==
  cfblk1 : Inport
  cfblk2 : Outport
  wires:
  cfblk1/1 -> cfblk2/1

== system sampleModel196/cfblk41/cfblk14/cfblk15/cfblk13 ==
  cfblk1 : Inport
  cfblk2 : Outport
  wires:
  cfblk1/1 -> cfblk2/1

== system sampleModel196/cfblk41/cfblk14/cfblk15/cfblk14 ==
  cfblk1 : Inport
  cfblk2 : Outport
  wires:
  cfblk1/1 -> cfblk2/1

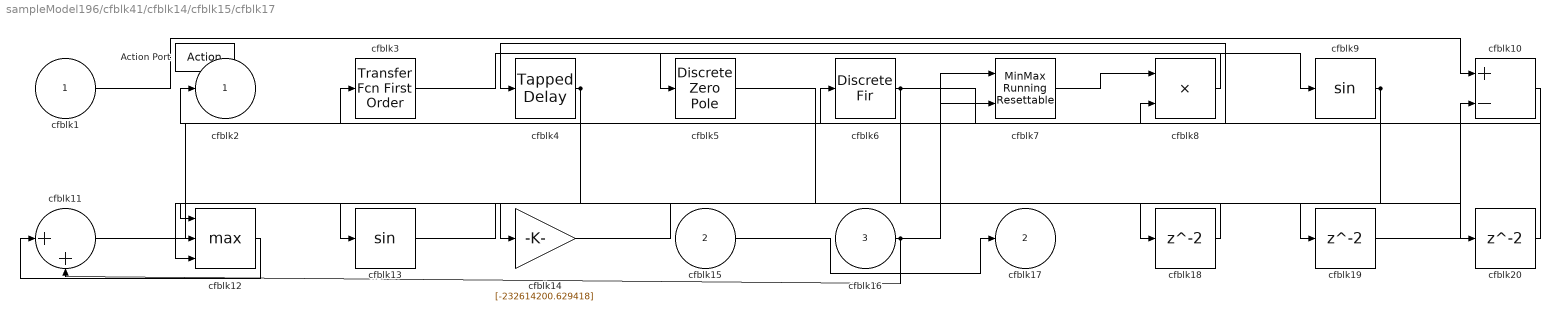
== system sampleModel196/cfblk41/cfblk14/cfblk15/cfblk17 ==
  cfblk1 : Inport
  cfblk15 : Inport  Port=2
  cfblk16 : Inport  Port=3
  Action Port : ActionPort  ActionType=then
  cfblk10 : Sum  Inputs=+-
  cfblk11 : Sum  Inputs=|++
  cfblk12 : MinMax  Function=max  Inputs=3
  cfblk13 : Trigonometry
  cfblk14 : Gain  Gain=[-232614200.629418]
  cfblk18 : Delay
  cfblk19 : Delay
  cfblk20 : Delay
  cfblk3 : simulink/Discrete/Transfer Fcn First Order  PoleZ=0.95  ICPrevOutput=0.0  DoSatur=off
      settings: SourceProductName=Simulink
  cfblk4 : simulink/Discrete/Tapped Delay  vinit=0.0  samptime=-1  NumDelays=1  DelayOrder=Oldest  includeCurrent=off
  cfblk5 : DiscreteZeroPole  Poles=[0 0.5]  Gain=1  SampleTime=-1
  cfblk6 : DiscreteFir
  cfblk7 : simulink/Math Operations/MinMax Running Resettable  Function=min  vinit=0.0
  cfblk8 : Product  Inputs=**
  cfblk9 : Trigonometry
  cfblk2 : Outport
  cfblk17 : Outport  Port=2
  wires:
  cfblk11/1 -> cfblk6/1
  cfblk12/1 -> cfblk11/1
  cfblk1/1 -> cfblk10/1
  cfblk6/1 -> cfblk14/1, cfblk7/2, cfblk8/2
  cfblk8/1 -> cfblk5/1
  cfblk10/1 -> cfblk4/1
  cfblk15/1 -> cfblk17/1
  cfblk9/1 -> cfblk13/1, cfblk12/3
  cfblk7/1 -> cfblk8/1
  cfblk16/1 -> cfblk11/2, cfblk7/1
  cfblk3/1 -> cfblk9/1
  cfblk4/1 -> cfblk12/2, cfblk2/1
  cfblk14/1 -> cfblk18/1
  cfblk18/1 -> cfblk12/1
  cfblk5/1 -> cfblk19/1
  cfblk19/1 -> cfblk10/2
  cfblk13/1 -> cfblk20/1
  cfblk20/1 -> cfblk3/1

== system sampleModel196/cfblk41/cfblk14/cfblk15/cfblk18 ==
  cfblk1 : Inport
  cfblk7 : Inport  Port=2
  Action Port : ActionPort  ActionType=else
  cfblk3 : DiscreteFir
  cfblk4 : Delay  DelayLengthSource=Input port
      settings: InputPortMap=u0,p1
  cfblk5 : ComplexToRealImag
  cfblk6 : Constant  Value=[21565379.290096]  SampleTime=1
  cfblk2 : Outport
  wires:
  cfblk7/1 -> cfblk5/1
  cfblk6/1 -> cfblk3/1
  cfblk1/1 -> cfblk4/1
  cfblk5/1 -> cfblk4/2
  cfblk5/2 -> cfblk2/1
